simulink model "Tread_carcass_Tire_thermal_model_simplified"  (R2024b)
settings: Solver=VariableStepAuto  StartTime=0  StopTime=2105  FixedStep=0.01  MaxStep=0.5  RelTol=1e-4
undefined symbols (not defined in the file): a_coeff, b_coeff, data, exponentialcoefficient_Fz, exponentialcoefficient_p, H_ta_constant, H_ta_proportional, H_tc, H_tread_road, M_tread, S_tread, TSTC, w_cp
settings Model: Creator=Utente  LastModifiedBy=Utente

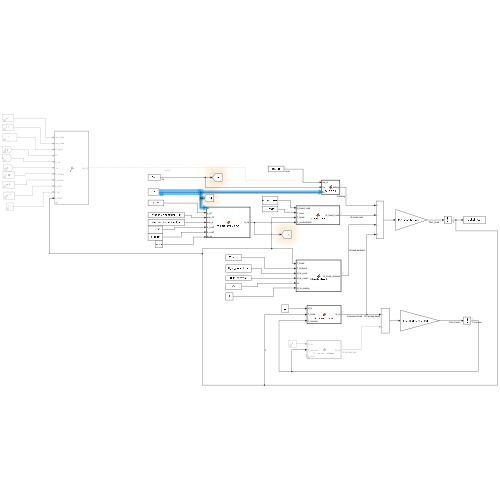
[thumbnail: Simulink's stored preview of the top-level diagram]
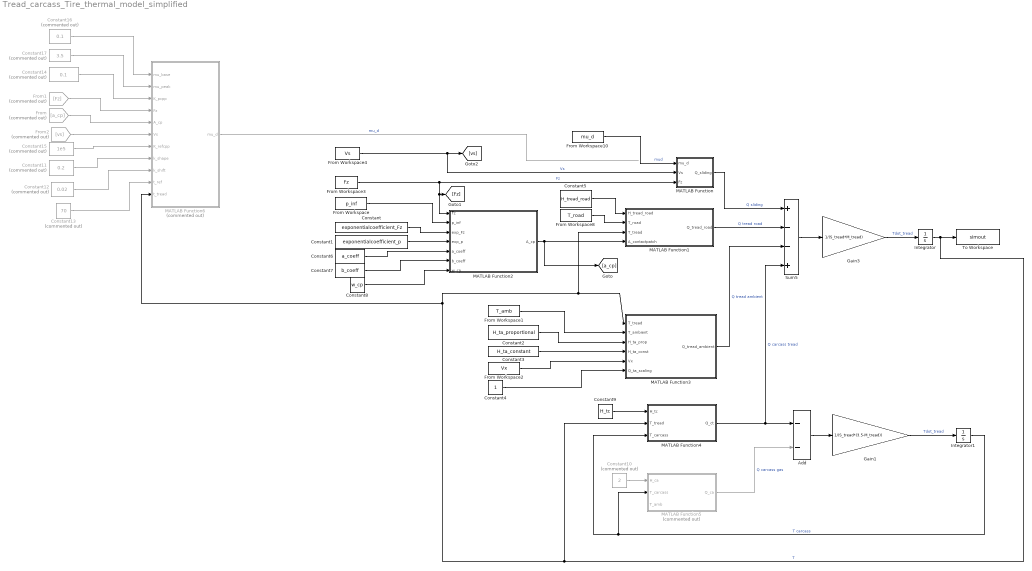
== system Tread_carcass_Tire_thermal_model_simplified ==
  Add : Sum  Inputs=--
  Constant : Constant  Value=exponentialcoefficient_Fz
  Constant1 : Constant  Value=exponentialcoefficient_p
  Constant10 : Constant  Commented=on  Value=2
  Constant11 : Constant  Commented=on  Value=0.2
  Constant12 : Constant  Commented=on  Value=0.02
  Constant13 : Constant  Commented=on  Value=70
  Constant14 : Constant  Commented=on  Value=0.1
  Constant15 : Constant  Commented=on  Value=1e5
  Constant16 : Constant  Commented=on  Value=0.1
  Constant17 : Constant  Commented=on  Value=3.5
  Constant2 : Constant  Value=H_ta_proportional
  Constant3 : Constant  Value=H_ta_constant
  Constant4 : Constant
  Constant5 : Constant  Value=H_tread_road
  Constant6 : Constant  Value=a_coeff
  Constant7 : Constant  Value=b_coeff
  Constant8 : Constant  Value=w_cp
  Constant9 : Constant  Value=H_tc
  From : From  Commented=on  GotoTag=a_cp
  From Workspace : FromWorkspace  VariableName=p_inf
  From Workspace1 : FromWorkspace  VariableName=T_amb
  From Workspace10 : FromWorkspace  VariableName=mu_d
  From Workspace2 : FromWorkspace  VariableName=Vx
  From Workspace3 : FromWorkspace  VariableName=Fz
  From Workspace4 : FromWorkspace  VariableName=Vs
  From Workspace8 : FromWorkspace  VariableName=T_road
  From1 : From  Commented=on  GotoTag=Fz
  From2 : From  Commented=on  GotoTag=vs
  Gain1 : Gain  Gain=1/(S_tread*(3.5-M_tread))
  Gain3 : Gain  Gain=1/(S_tread*M_tread)
  Integrator : Integrator  InitialCondition=data.TSTC(1)
  Integrator1 : Integrator  InitialCondition=TSTC(1)
  MATLAB Function : MATLAB Function  TreatAsAtomicUnit=on
  MATLAB Function1 : MATLAB Function  TreatAsAtomicUnit=on
  MATLAB Function2 : MATLAB Function  TreatAsAtomicUnit=on
  MATLAB Function3 : MATLAB Function  TreatAsAtomicUnit=on
  MATLAB Function4 : MATLAB Function  TreatAsAtomicUnit=on
  MATLAB Function5 : MATLAB Function  Commented=on  TreatAsAtomicUnit=on
  MATLAB Function6 : MATLAB Function  Commented=on  TreatAsAtomicUnit=on
  Sum5 : Sum  Inputs=+--+
  To Workspace : ToWorkspace  VariableName=simout  SaveFormat=Timeseries  SampleTime=-1
  wires:
  Gain3/1 -> Integrator/1  "Tdot_tread"
  From Workspace4/1 -> MATLAB Function/2(Vs), [vs]  "Vs"
  Sum5/1 -> Gain3/1
  Integrator/1 -> To Workspace/1, MATLAB Function4/2(T_tread), MATLAB Function6/11(t_tread), MATLAB Function1/3(T_tread), MATLAB Function3/1(T_tread)  "T"
  MATLAB Function/1(Q_sliding) -> Sum5/1  "Q sliding"
  From Workspace3/1 -> [Fz], MATLAB Function2/1(Fz), MATLAB Function/3(Fz)  "Fz"
  Constant5/1 -> MATLAB Function1/1(H_tread_road)
  MATLAB Function1/1(Q_tread_road) -> Sum5/2  "Q tread road"
  From Workspace8/1 -> MATLAB Function1/2(T_road)
  Constant1/1 -> MATLAB Function2/4(exp_p)
  Constant/1 -> MATLAB Function2/3(exp_Fz)
  Constant6/1 -> MATLAB Function2/5(a_coeff)
  Constant7/1 -> MATLAB Function2/6(b_coeff)
  Constant8/1 -> MATLAB Function2/7(w_cp)
  From Workspace/1 -> MATLAB Function2/2(p_inf)
  MATLAB Function2/1(A_cp) -> [a_cp], MATLAB Function1/4(A_contactpatch)
  Constant2/1 -> MATLAB Function3/3(H_ta_prop)
  Constant3/1 -> MATLAB Function3/4(H_ta_const)
  From Workspace2/1 -> MATLAB Function3/5(Vx)
  From Workspace1/1 -> MATLAB Function3/2(T_ambient)
  Constant4/1 -> MATLAB Function3/6(Q_ta_scaling)
  MATLAB Function3/1(Q_tread_ambient) -> Sum5/3  "Q tread ambient"
  MATLAB Function4/1(Q_ct) -> Add/1, Sum5/4  "Q carcass tread"
  Integrator1/1 -> MATLAB Function5/2(T_carcass), MATLAB Function4/3(T_carcass)  "T carcass"
  Gain1/1 -> Integrator1/1  "Tdot_tread"
  Constant9/1 -> MATLAB Function4/1(H_tc)
  Constant10/1 -> MATLAB Function5/1(H_ca)
  Add/1 -> Gain1/1
  MATLAB Function5/1(Q_ca) -> Add/2  "Q carcass gas"
  Constant16/1 -> MATLAB Function6/1(mu_base)
  Constant17/1 -> MATLAB Function6/2(mu_peak)
  Constant14/1 -> MATLAB Function6/3(K_pcpp)
  From1/1 -> MATLAB Function6/4(Fz)
  From/1 -> MATLAB Function6/5(A_cp)
  From2/1 -> MATLAB Function6/6(Vs)
  Constant15/1 -> MATLAB Function6/7(K_refcpp)
  Constant11/1 -> MATLAB Function6/8(k_shape)
  Constant12/1 -> MATLAB Function6/9(k_shift)
  Constant13/1 -> MATLAB Function6/10(t_ref)
  MATLAB Function6/1(mu_d) -> ?  "mu_d"
  From Workspace10/1 -> MATLAB Function/1(mu_d)  "mud"

== matlab function Tread_carcass_Tire_thermal_model_simplified/MATLAB Function1 ==
  data: H_tread_road input; T_road input; T_tread input; Q_tread_road output; A_contactpatch input
function Q_tread_road = Q_tread_road(H_tread_road,T_road, T_tread, A_contactpatch)

Q_tread_road = H_tread_road*A_contactpatch*(T_tread-T_road);
end

== matlab function Tread_carcass_Tire_thermal_model_simplified/MATLAB Function ==
  data: mu_d input; Vs input; Q_sliding output; Fz input
function Q_sliding = Q_sliding(mu_d, Vs, Fz)

Q_sliding = mu_d*Fz*Vs;

end

== matlab function Tread_carcass_Tire_thermal_model_simplified/MATLAB Function2 ==
  data: Fz input; p_inf input; exp_Fz input; A_cp output; exp_p input; a_coeff input; b_coeff input; w_cp input
function A_cp = contact_patch_area(Fz, p_inf, exp_Fz, exp_p,a_coeff, b_coeff, w_cp)

%af2 = (a_coeff*p_inf^(-exp_p))*(abs(Fz)/b_coeff)^exp_Fz;
% Prevent zero or negative values in p_inf and Fz
p_inf(p_inf <= 0) = 1e-6;  % Avoid zero/negative exponentiation
Fz(Fz == 0) = 1e-2;        % Avoid division by zero

% Compute af2 safely
af2 = (a_coeff * p_inf.^(-exp_p)) .* (max(abs(Fz), 1e-6) ./ b_coeff).^exp_Fz;

% Check for NaN or Inf
if any(isnan(af2(:))) || any(isinf(af2(:)))
    error('Error: NaN or Inf detected in af2 calculation!');
end

A_cp = af2*w_cp;

end

== matlab function Tread_carcass_Tire_thermal_model_simplified/MATLAB Function3 ==
  data: T_tread input; T_ambient input; H_ta_prop input; H_ta_const input; Q_tread_ambient output; Vx input; Q_ta_scaling input
function Q_tread_ambient = Qtreadambient(T_tread, T_ambient,H_ta_prop, H_ta_const, Vx,  Q_ta_scaling)

Q_tread_ambient = Q_ta_scaling*(H_ta_prop*Vx + H_ta_const)*(T_tread - T_ambient);

end

== matlab function Tread_carcass_Tire_thermal_model_simplified/MATLAB Function4 ==
  data: H_tc input; T_tread input; Q_ct output; T_carcass input
function Q_ct = Q_carcass_tread(H_tc, T_tread, T_carcass)

Q_ct =  H_tc.*(T_carcass - T_tread);

end

== matlab function Tread_carcass_Tire_thermal_model_simplified/MATLAB Function5 ==
  data: H_ca input; T_carcass input; T_amb input; Q_ca output
function Q_ca = Q_carcass_ambient(H_ca, T_carcass, T_amb)

Q_ca =  H_ca.*(T_carcass - T_amb);

end

== matlab function Tread_carcass_Tire_thermal_model_simplified/MATLAB Function6 ==
  data: mu_base input; mu_d output; mu_peak input; K_pcpp input; Fz input; A_cp input; Vs input; K_refcpp input; k_shape input; k_shift input; t_ref input; t_tread input
% function mu_d = fcn(mu_base, mu_peak, K_pcpp, Fz, A_cp,Vs, K_refcpp, k_shape, k_shift, t_ref, t_tread)
% 
% P_cp = Fz/A_cp;
% kcpp = 1 - K_pcpp*P_cp/K_refcpp;
% %mu_mc = mu_base + (mu_peak - mu_base)*exp(-k_shape*(log10(Vs) - k_shift*(t_tread - t_ref)))^2;
% mu_mc = mu_base + (mu_peak - mu_base) * exp((-k_shape * (log10(Vs) - k_shift * (t_tread - t_ref)))^2);
% 
% mu_d = kcpp*mu_mc;
% 
% end

function mu_d = fcn(mu_base, mu_peak, K_pcpp, Fz, A_cp, Vs, K_refcpp, k_shape, k_shift, t_ref, t_tread)

    % Avoid division by zero in A_cp
    P_cp = Fz / max(A_cp, 1e-6);
    
    % Compute kcpp
    kcpp = 1 - K_pcpp * P_cp / K_refcpp;
    
    % Ensure Vs is not zero to avoid log(0)
    Vs = max(Vs, 1e-6);
    
    % Compute mu_mc with correct exponentiation
    mu_mc = mu_base + (mu_peak - mu_base) * exp((-k_shape * (log10(Vs) - k_shift * (t_tread - t_ref)))^2);
    
    % Compute final mu_d
    mu_d = kcpp * mu_mc;

end
